simulink library "ammclib_bam_s32k14x"  (Simulink 9.0)
settings: Solver=ode45  StartTime=0.0  StopTime=10.0  RelTol=1e-3
undefined symbols (not defined in the file): f16A1, f16A2, f16B0, f16B1, f16B2, f16C1, f16CC1, f16CC1sc, f16CC1sc_D, f16CC1sc_Q, f16CC1scD, f16CC1scQ, f16CC2, f16CC2sc, f16CC2sc_D, f16CC2sc_Q, f16CC2scD, f16CC2scQ, f16DerivGain, f16EGain, f16FiltCoef, f16HystOff, f16HystOn, f16IGain, f16IntegGain, f16IntegGainFW, f16IntegGainQ, f16Kd, f16Kq, f16Limit, f16LowerLim, f16LowerLimit_D, f16LowerLimit_Q, f16ModIndex, f16OutValOff, f16OutValOn, f16PropGain, f16PropGainFW, f16PropGainQ, f16RampDown, f16RampUp, f16UGain, f16UpperLim, f16UpperLimit, f16UpperLimit_D, f16UpperLimit_Q, f16WIGain, f32A1, f32A2, f32B0, f32B1, f32B2, f32C1, f32CC1, f32CC1sc, f32CC1sc_D, f32CC1sc_Q, f32CC1scD, f32CC1scQ, f32CC2 ... (+122)
(part 5 of 11)

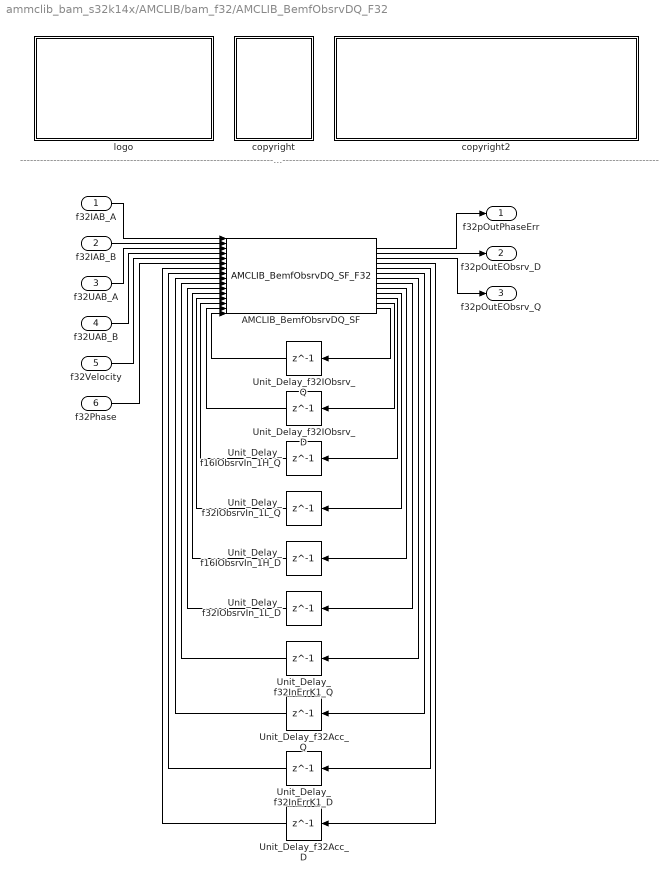
== system ammclib_bam_s32k14x/AMCLIB/bam_f32/AMCLIB_BemfObsrvDQ_F32 ==
  note: ---------------------------------------------------------------------------------------------------------------------------------------------------------------------------------------------------
  f32IAB_A : Inport
  f32IAB_B : Inport  Port=2
  f32UAB_A : Inport  Port=3
  f32UAB_B : Inport  Port=4
  f32Velocity : Inport  Port=5
  f32Phase : Inport  Port=6
  AMCLIB_BemfObsrvDQ_SF : S-Function  FunctionName=AMCLIB_BemfObsrvDQ_SF_F32  Parameters=f32IGain,f32UGain,f32WIGain,f32EGain,s16Shift,f32CC1sc_D,f32CC1sc_Q,f32CC2sc_D,f32CC2sc_Q,f32UpperLimit_D,f32UpperLimit_Q,f32LowerLimit_D,f32LowerLimit_Q,u16NShift  SFunctionDeploymentMode=off  EnableBusSupport=off
  Unit_Delay_f16IObsrvIn_1H_D : Delay  DelayLength=1  InitialCondition=0
  Unit_Delay_f16IObsrvIn_1H_Q : Delay  DelayLength=1  InitialCondition=0
  Unit_Delay_f32Acc_D : Delay  DelayLength=1  InitialCondition=0
  Unit_Delay_f32Acc_Q : Delay  DelayLength=1  InitialCondition=0
  Unit_Delay_f32IObsrvIn_1L_D : Delay  DelayLength=1  InitialCondition=0
  Unit_Delay_f32IObsrvIn_1L_Q : Delay  DelayLength=1  InitialCondition=0
  Unit_Delay_f32IObsrv_D : Delay  DelayLength=1  InitialCondition=0
  Unit_Delay_f32IObsrv_Q : Delay  DelayLength=1  InitialCondition=0
  Unit_Delay_f32InErrK1_D : Delay  DelayLength=1  InitialCondition=0
  Unit_Delay_f32InErrK1_Q : Delay  DelayLength=1  InitialCondition=0
  copyright : Subsystem
      mask Display: text(10,90,'FILE:');text(10,75,'DESRIPTION:');text(10,60,'COPYRIGHT:');text(10,45,'VERSION:');text(10,30,'DATE:')
  copyright2 : Subsystem
      mask Display: text(10,90,'AMCLIB_BemfObsrvDQ_BAM_F32.mdl');text(10,75,'PMSM back-EMF observer DQ.');text(10,60,'NXP');text(10,45,'1.0');text(10,30,'26-Oct-2016');
  logo : Subsystem
      mask Display: image(imread('logo.jpg'))
  f32pOutPhaseErr : Outport
  f32pOutEObsrv_D : Outport  Port=2
  f32pOutEObsrv_Q : Outport  Port=3
  wires:
  AMCLIB_BemfObsrvDQ_SF/3 -> f32pOutEObsrv_Q/1
  AMCLIB_BemfObsrvDQ_SF/2 -> f32pOutEObsrv_D/1
  AMCLIB_BemfObsrvDQ_SF/1 -> f32pOutPhaseErr/1
  f32Phase/1 -> AMCLIB_BemfObsrvDQ_SF/6
  f32Velocity/1 -> AMCLIB_BemfObsrvDQ_SF/5
  f32UAB_B/1 -> AMCLIB_BemfObsrvDQ_SF/4
  f32UAB_A/1 -> AMCLIB_BemfObsrvDQ_SF/3
  f32IAB_B/1 -> AMCLIB_BemfObsrvDQ_SF/2
  f32IAB_A/1 -> AMCLIB_BemfObsrvDQ_SF/1
  Unit_Delay_f32IObsrv_Q/1 -> AMCLIB_BemfObsrvDQ_SF/16
  Unit_Delay_f32IObsrv_D/1 -> AMCLIB_BemfObsrvDQ_SF/15
  Unit_Delay_f16IObsrvIn_1H_Q/1 -> AMCLIB_BemfObsrvDQ_SF/14
  AMCLIB_BemfObsrvDQ_SF/13 -> Unit_Delay_f32IObsrv_Q/1
  AMCLIB_BemfObsrvDQ_SF/12 -> Unit_Delay_f32IObsrv_D/1
  AMCLIB_BemfObsrvDQ_SF/11 -> Unit_Delay_f16IObsrvIn_1H_Q/1
  AMCLIB_BemfObsrvDQ_SF/10 -> Unit_Delay_f32IObsrvIn_1L_Q/1
  Unit_Delay_f32IObsrvIn_1L_Q/1 -> AMCLIB_BemfObsrvDQ_SF/13
  Unit_Delay_f16IObsrvIn_1H_D/1 -> AMCLIB_BemfObsrvDQ_SF/12
  AMCLIB_BemfObsrvDQ_SF/9 -> Unit_Delay_f16IObsrvIn_1H_D/1
  AMCLIB_BemfObsrvDQ_SF/8 -> Unit_Delay_f32IObsrvIn_1L_D/1
  Unit_Delay_f32IObsrvIn_1L_D/1 -> AMCLIB_BemfObsrvDQ_SF/11
  Unit_Delay_f32InErrK1_Q/1 -> AMCLIB_BemfObsrvDQ_SF/10
  AMCLIB_BemfObsrvDQ_SF/7 -> Unit_Delay_f32InErrK1_Q/1
  AMCLIB_BemfObsrvDQ_SF/6 -> Unit_Delay_f32Acc_Q/1
  Unit_Delay_f32Acc_Q/1 -> AMCLIB_BemfObsrvDQ_SF/9
  Unit_Delay_f32InErrK1_D/1 -> AMCLIB_BemfObsrvDQ_SF/8
  Unit_Delay_f32Acc_D/1 -> AMCLIB_BemfObsrvDQ_SF/7
  AMCLIB_BemfObsrvDQ_SF/5 -> Unit_Delay_f32InErrK1_D/1
  AMCLIB_BemfObsrvDQ_SF/4 -> Unit_Delay_f32Acc_D/1

== system ammclib_bam_s32k14x/AMCLIB/bam_f32/AMCLIB_CurrentLoop_F32 ==
  note: ---------------------------------------------------------------------------------------------------------------------------------------------------------------------------------------------------
  f32UDcBus : Inport
  f32IDReq : Inport  Port=2
  f32IQReq : Inport  Port=3
  f32IDFbck : Inport  Port=4
  f32IQFbck : Inport  Port=5
  AMCLIB_CurrentLoop_SF : S-Function  FunctionName=AMCLIB_CurrentLoop_SF_F32  Parameters=f32CC1scD,f32CC2scD,u16NShiftD,f32CC1scQ,f32CC2scQ,u16NShiftQ  SFunctionDeploymentMode=off  EnableBusSupport=off
  Delay{30..33} (4 alike) : Delay  DelayLength=1  InitialCondition=0
  copyright : Subsystem
      mask Display: text(10,90,'FILE:');text(10,75,'DESRIPTION:');text(10,60,'COPYRIGHT:');text(10,45,'VERSION:');text(10,30,'DATE:')
  copyright2 : Subsystem
      mask Display: text(10,90,'AMCLIB_CurrentLoop_BAM_F32.mdl');text(10,75,'PMSM Current Loop.');text(10,60,'NXP');text(10,45,'1.0');text(10,30,'25-Oct-2017');
  logo : Subsystem
      mask Display: image(imread('logo.jpg'))
  pOutUDReq : Outport
  pOutUQReq : Outport  Port=2
  wires:
  f32UDcBus/1 -> AMCLIB_CurrentLoop_SF/1
  f32IDReq/1 -> AMCLIB_CurrentLoop_SF/2
  f32IQReq/1 -> AMCLIB_CurrentLoop_SF/3
  f32IDFbck/1 -> AMCLIB_CurrentLoop_SF/4
  f32IQFbck/1 -> AMCLIB_CurrentLoop_SF/5
  Delay32/1 -> AMCLIB_CurrentLoop_SF/6
  Delay31/1 -> AMCLIB_CurrentLoop_SF/7
  Delay30/1 -> AMCLIB_CurrentLoop_SF/8
  Delay33/1 -> AMCLIB_CurrentLoop_SF/9
  AMCLIB_CurrentLoop_SF/1 -> Delay32/1
  AMCLIB_CurrentLoop_SF/2 -> Delay31/1
  AMCLIB_CurrentLoop_SF/3 -> Delay30/1
  AMCLIB_CurrentLoop_SF/4 -> Delay33/1
  AMCLIB_CurrentLoop_SF/5 -> pOutUDReq/1
  AMCLIB_CurrentLoop_SF/6 -> pOutUQReq/1

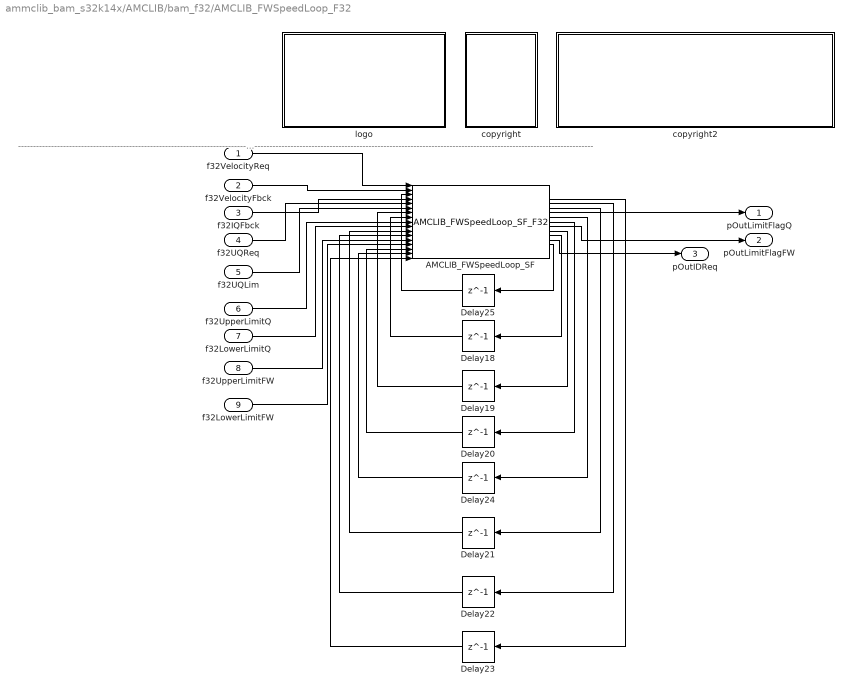
== system ammclib_bam_s32k14x/AMCLIB/bam_f32/AMCLIB_FWSpeedLoop_F32 ==
  note: ---------------------------------------------------------------------------------------------------------------------------------------------------------------------------------------------------
  f32VelocityReq : Inport
  f32VelocityFbck : Inport  Port=2
  f32IQFbck : Inport  Port=3
  f32UQReq : Inport  Port=4
  f32UQLim : Inport  Port=5
  f32UpperLimitQ : Inport  Port=6
  f32LowerLimitQ : Inport  Port=7
  f32UpperLimitFW : Inport  Port=8
  f32LowerLimitFW : Inport  Port=9
  AMCLIB_FWSpeedLoop_SF : S-Function  FunctionName=AMCLIB_FWSpeedLoop_SF_F32  Parameters=u16NSamplesW,u16NSamplesFW,f32PropGainQ,s16PropGainShiftQ,f32IntegGainQ,s16IntegGainShiftQ,f32PropGainFW,s16PropGainShiftFW,f32IntegGainFW,s16IntegGainShiftFW,f32RampUp,f32RampDown  SFunctionDeploymentMode=off  EnableBusSupport=off
  Delay{18..25} (8 alike) : Delay  DelayLength=1  InitialCondition=0
  copyright : Subsystem
      mask Display: text(10,90,'FILE:');text(10,75,'DESRIPTION:');text(10,60,'COPYRIGHT:');text(10,45,'VERSION:');text(10,30,'DATE:')
  copyright2 : Subsystem
      mask Display: text(10,90,'AMCLIB_FWSpeedLoop_BAM_F32.mdl');text(10,75,'Speed Loop with Field Weakening.');text(10,60,'NXP');text(10,45,'1.0');text(10,30,'28-Aug-2017');
  logo : Subsystem
      mask Display: image(imread('logo.jpg'))
  pOutLimitFlagQ : Outport
  pOutLimitFlagFW : Outport  Port=2
  pOutIDReq : Outport  Port=3
  wires:
  f32VelocityReq/1 -> AMCLIB_FWSpeedLoop_SF/1
  f32VelocityFbck/1 -> AMCLIB_FWSpeedLoop_SF/2
  Delay25/1 -> AMCLIB_FWSpeedLoop_SF/3
  f32IQFbck/1 -> AMCLIB_FWSpeedLoop_SF/4
  f32UQReq/1 -> AMCLIB_FWSpeedLoop_SF/5
  f32UQLim/1 -> AMCLIB_FWSpeedLoop_SF/6
  Delay19/1 -> AMCLIB_FWSpeedLoop_SF/7
  Delay18/1 -> AMCLIB_FWSpeedLoop_SF/8
  f32UpperLimitQ/1 -> AMCLIB_FWSpeedLoop_SF/9
  f32LowerLimitQ/1 -> AMCLIB_FWSpeedLoop_SF/10
  Delay21/1 -> AMCLIB_FWSpeedLoop_SF/11
  Delay22/1 -> AMCLIB_FWSpeedLoop_SF/12
  f32UpperLimitFW/1 -> AMCLIB_FWSpeedLoop_SF/13
  f32LowerLimitFW/1 -> AMCLIB_FWSpeedLoop_SF/14
  Delay20/1 -> AMCLIB_FWSpeedLoop_SF/15
  Delay24/1 -> AMCLIB_FWSpeedLoop_SF/16
  Delay23/1 -> AMCLIB_FWSpeedLoop_SF/17
  AMCLIB_FWSpeedLoop_SF/1 -> Delay23/1
  AMCLIB_FWSpeedLoop_SF/2 -> Delay22/1
  AMCLIB_FWSpeedLoop_SF/3 -> Delay21/1
  AMCLIB_FWSpeedLoop_SF/4 -> pOutLimitFlagQ/1
  AMCLIB_FWSpeedLoop_SF/5 -> Delay24/1
  AMCLIB_FWSpeedLoop_SF/6 -> Delay20/1
  AMCLIB_FWSpeedLoop_SF/7 -> pOutLimitFlagFW/1
  AMCLIB_FWSpeedLoop_SF/8 -> Delay19/1
  AMCLIB_FWSpeedLoop_SF/9 -> Delay18/1
  AMCLIB_FWSpeedLoop_SF/10 -> pOutIDReq/1
  AMCLIB_FWSpeedLoop_SF/11 -> Delay25/1

== system ammclib_bam_s32k14x/AMCLIB/bam_f32/AMCLIB_FW_F32 ==
  note: ---------------------------------------------------------------------------------------------------------------------------------------------------------------------------------------------------
  f32ReqAmp : Inport
  f32VelocityFbck : Inport  Port=2
  f32IQFbck : Inport  Port=3
  f32UQReq : Inport  Port=4
  f32UQLim : Inport  Port=5
  f32UpperLimitFW : Inport  Port=6
  f32LowerLimitFW : Inport  Port=7
  AMCLIB_FW_SF : S-Function  FunctionName=AMCLIB_FW_SF_F32  Parameters=u16NSamplesFW,f32PropGainFW,s16PropGainShiftFW,f32IntegGainFW,s16IntegGainShiftFW  SFunctionDeploymentMode=off  EnableBusSupport=off
  Delay{26..29} (4 alike) : Delay  DelayLength=1  InitialCondition=0
  copyright : Subsystem
      mask Display: text(10,90,'FILE:');text(10,75,'DESRIPTION:');text(10,60,'COPYRIGHT:');text(10,45,'VERSION:');text(10,30,'DATE:')
  copyright2 : Subsystem
      mask Display: text(10,90,'AMCLIB_FW_BAM_F32.mdl');text(10,75,'Speed Loop with Field Weakening.');text(10,60,'NXP');text(10,45,'1.0');text(10,30,'28-Aug-2017');
  logo : Subsystem
      mask Display: image(imread('logo.jpg'))
  pOutLimitFlagFW : Outport
  pOutIDReq : Outport  Port=2
  wires:
  f32ReqAmp/1 -> AMCLIB_FW_SF/1
  f32VelocityFbck/1 -> AMCLIB_FW_SF/2
  Delay29/1 -> AMCLIB_FW_SF/3
  f32IQFbck/1 -> AMCLIB_FW_SF/4
  f32UQReq/1 -> AMCLIB_FW_SF/5
  f32UQLim/1 -> AMCLIB_FW_SF/6
  Delay26/1 -> AMCLIB_FW_SF/7
  f32UpperLimitFW/1 -> AMCLIB_FW_SF/8
  f32LowerLimitFW/1 -> AMCLIB_FW_SF/9
  Delay27/1 -> AMCLIB_FW_SF/10
  Delay28/1 -> AMCLIB_FW_SF/11
  AMCLIB_FW_SF/1 -> Delay28/1
  AMCLIB_FW_SF/2 -> Delay27/1
  AMCLIB_FW_SF/3 -> pOutLimitFlagFW/1
  AMCLIB_FW_SF/4 -> Delay26/1
  AMCLIB_FW_SF/5 -> pOutIDReq/1
  AMCLIB_FW_SF/6 -> Delay29/1

== system ammclib_bam_s32k14x/AMCLIB/bam_f32/AMCLIB_SpeedLoop_F32 ==
  note: ---------------------------------------------------------------------------------------------------------------------------------------------------------------------------------------------------
  f32VelocityReq : Inport
  f32VelocityFbck : Inport  Port=2
  f32UpperLimitQ : Inport  Port=3
  f32LowerLimitQ : Inport  Port=4
  AMCLIB_SpeedLoop_SF : S-Function  FunctionName=AMCLIB_SpeedLoop_SF_F32  Parameters=u16NSamplesW,f32PropGainQ,s16PropGainShiftQ,f32IntegGainQ,s16IntegGainShiftQ,f32RampUp,f32RampDown  SFunctionDeploymentMode=off  EnableBusSupport=off
  Delay{1,14..15,17} (4 alike) : Delay  DelayLength=1  InitialCondition=0
  copyright : Subsystem
      mask Display: text(10,90,'FILE:');text(10,75,'DESRIPTION:');text(10,60,'COPYRIGHT:');text(10,45,'VERSION:');text(10,30,'DATE:')
  copyright2 : Subsystem
      mask Display: text(10,90,'AMCLIB_SpeedLoop_BAM_F32.mdl');text(10,75,'Speed Loop with Field Weakening.');text(10,60,'NXP');text(10,45,'1.0');text(10,30,'28-Aug-2017');
  logo : Subsystem
      mask Display: image(imread('logo.jpg'))
  pOutLimitFlagQ : Outport
  pOutIQReq : Outport  Port=2
  wires:
  f32VelocityReq/1 -> AMCLIB_SpeedLoop_SF/1
  f32VelocityFbck/1 -> AMCLIB_SpeedLoop_SF/2
  Delay17/1 -> AMCLIB_SpeedLoop_SF/3
  f32UpperLimitQ/1 -> AMCLIB_SpeedLoop_SF/4
  f32LowerLimitQ/1 -> AMCLIB_SpeedLoop_SF/5
  Delay14/1 -> AMCLIB_SpeedLoop_SF/6
  Delay15/1 -> AMCLIB_SpeedLoop_SF/7
  Delay1/1 -> AMCLIB_SpeedLoop_SF/8
  AMCLIB_SpeedLoop_SF/1 -> Delay1/1
  AMCLIB_SpeedLoop_SF/2 -> Delay15/1
  AMCLIB_SpeedLoop_SF/3 -> Delay14/1
  AMCLIB_SpeedLoop_SF/4 -> pOutLimitFlagQ/1
  AMCLIB_SpeedLoop_SF/5 -> Delay17/1
  AMCLIB_SpeedLoop_SF/6 -> pOutIQReq/1

== system ammclib_bam_s32k14x/AMCLIB/bam_f32/AMCLIB_TrackObsrv_F32 ==
  note: ---------------------------------------------------------------------------------------------------------------------------------------------------------------------------------------------------
  f32PhaseErr : Inport
  f32UpperLimit : Inport  Port=2
  f32LowerLimit : Inport  Port=3
  AMCLIB_TrackObsrv_SF : S-Function  FunctionName=AMCLIB_TrackObsrv_SF_F32  Parameters=f32CC1sc,f32CC2sc,u16NShift,f32C1,u16IntegNShift  SFunctionDeploymentMode=off  EnableBusSupport=off
  Unit_Delay_f32Acc : Delay  DelayLength=1  InitialCondition=0
  Unit_Delay_f32InErrK1 : Delay  DelayLength=1  InitialCondition=0
  Unit_Delay_f32InK1 : Delay  DelayLength=1  InitialCondition=0
  Unit_Delay_f32State : Delay  DelayLength=1  InitialCondition=0
  copyright : Subsystem
      mask Display: text(10,90,'FILE:');text(10,75,'DESRIPTION:');text(10,60,'COPYRIGHT:');text(10,45,'VERSION:');text(10,30,'DATE:')
  copyright2 : Subsystem
      mask Display: text(10,90,'AMCLIB_TrackObsrv_BAM_F32.mdl');text(10,75,'Tracking observer function.');text(10,60,'NXP');text(10,45,'1.0');text(10,30,'29-Jul-2016');
  logo : Subsystem
      mask Display: image(imread('logo.jpg'))
  f32PosEst : Outport
  f32VelocityEst : Outport  Port=2
  wires:
  AMCLIB_TrackObsrv_SF/2 -> f32VelocityEst/1
  AMCLIB_TrackObsrv_SF/1 -> f32PosEst/1
  f32LowerLimit/1 -> AMCLIB_TrackObsrv_SF/5
  f32UpperLimit/1 -> AMCLIB_TrackObsrv_SF/4
  f32PhaseErr/1 -> AMCLIB_TrackObsrv_SF/1
  Unit_Delay_f32InK1/1 -> AMCLIB_TrackObsrv_SF/7
  AMCLIB_TrackObsrv_SF/6 -> Unit_Delay_f32InK1/1
  Unit_Delay_f32State/1 -> AMCLIB_TrackObsrv_SF/6
  AMCLIB_TrackObsrv_SF/5 -> Unit_Delay_f32State/1
  Unit_Delay_f32InErrK1/1 -> AMCLIB_TrackObsrv_SF/3
  Unit_Delay_f32Acc/1 -> AMCLIB_TrackObsrv_SF/2
  AMCLIB_TrackObsrv_SF/4 -> Unit_Delay_f32InErrK1/1
  AMCLIB_TrackObsrv_SF/3 -> Unit_Delay_f32Acc/1

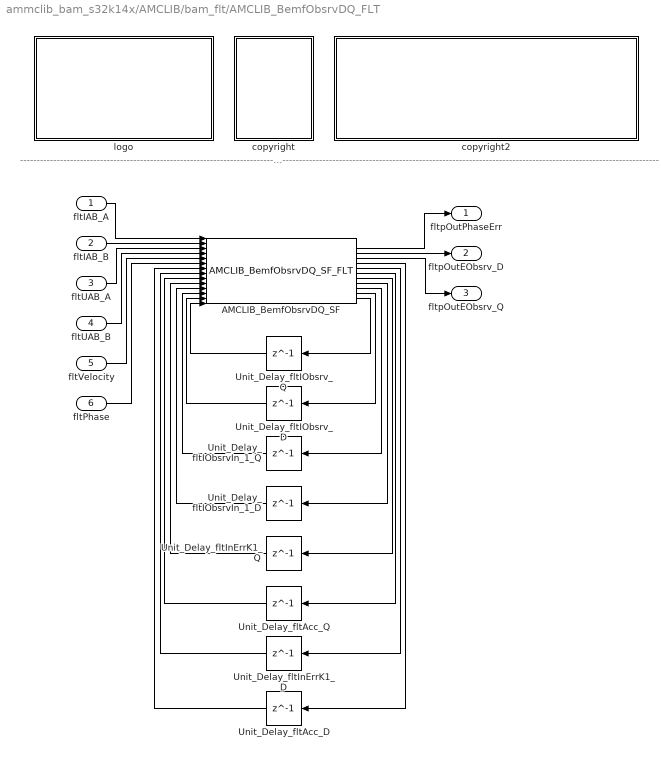
== system ammclib_bam_s32k14x/AMCLIB/bam_flt/AMCLIB_BemfObsrvDQ_FLT ==
  note: ---------------------------------------------------------------------------------------------------------------------------------------------------------------------------------------------------
  fltIAB_A : Inport
  fltIAB_B : Inport  Port=2
  fltUAB_A : Inport  Port=3
  fltUAB_B : Inport  Port=4
  fltVelocity : Inport  Port=5
  fltPhase : Inport  Port=6
  AMCLIB_BemfObsrvDQ_SF : S-Function  FunctionName=AMCLIB_BemfObsrvDQ_SF_FLT  Parameters=fltIGain,fltUGain,fltWIGain,fltEGain,fltCC1sc_D,fltCC1sc_Q,fltCC2sc_D,fltCC2sc_Q,fltUpperLimit_D,fltUpperLimit_Q,fltLowerLimit_D,fltLowerLimit_Q  SFunctionDeploymentMode=off  EnableBusSupport=off
  Unit_Delay_fltAcc_D : Delay  DelayLength=1  InitialCondition=0
  Unit_Delay_fltAcc_Q : Delay  DelayLength=1  InitialCondition=0
  Unit_Delay_fltIObsrvIn_1_D : Delay  DelayLength=1  InitialCondition=0
  Unit_Delay_fltIObsrvIn_1_Q : Delay  DelayLength=1  InitialCondition=0
  Unit_Delay_fltIObsrv_D : Delay  DelayLength=1  InitialCondition=0
  Unit_Delay_fltIObsrv_Q : Delay  DelayLength=1  InitialCondition=0
  Unit_Delay_fltInErrK1_D : Delay  DelayLength=1  InitialCondition=0
  Unit_Delay_fltInErrK1_Q : Delay  DelayLength=1  InitialCondition=0
  copyright : Subsystem
      mask Display: text(10,90,'FILE:');text(10,75,'DESRIPTION:');text(10,60,'COPYRIGHT:');text(10,45,'VERSION:');text(10,30,'DATE:')
  copyright2 : Subsystem
      mask Display: text(10,90,'AMCLIB_BemfObsrvDQ_BAM_FLT.mdl');text(10,75,'PMSM back-EMF observer DQ.');text(10,60,'NXP');text(10,45,'1.0');text(10,30,'26-Oct-2016');
  logo : Subsystem
      mask Display: image(imread('logo.jpg'))
  fltpOutPhaseErr : Outport
  fltpOutEObsrv_D : Outport  Port=2
  fltpOutEObsrv_Q : Outport  Port=3
  wires:
  AMCLIB_BemfObsrvDQ_SF/3 -> fltpOutEObsrv_Q/1
  AMCLIB_BemfObsrvDQ_SF/2 -> fltpOutEObsrv_D/1
  AMCLIB_BemfObsrvDQ_SF/1 -> fltpOutPhaseErr/1
  fltPhase/1 -> AMCLIB_BemfObsrvDQ_SF/6
  fltVelocity/1 -> AMCLIB_BemfObsrvDQ_SF/5
  fltUAB_B/1 -> AMCLIB_BemfObsrvDQ_SF/4
  fltUAB_A/1 -> AMCLIB_BemfObsrvDQ_SF/3
  fltIAB_B/1 -> AMCLIB_BemfObsrvDQ_SF/2
  fltIAB_A/1 -> AMCLIB_BemfObsrvDQ_SF/1
  Unit_Delay_fltIObsrv_Q/1 -> AMCLIB_BemfObsrvDQ_SF/14
  Unit_Delay_fltIObsrv_D/1 -> AMCLIB_BemfObsrvDQ_SF/13
  Unit_Delay_fltIObsrvIn_1_Q/1 -> AMCLIB_BemfObsrvDQ_SF/12
  Unit_Delay_fltIObsrvIn_1_D/1 -> AMCLIB_BemfObsrvDQ_SF/11
  Unit_Delay_fltInErrK1_Q/1 -> AMCLIB_BemfObsrvDQ_SF/10
  Unit_Delay_fltAcc_Q/1 -> AMCLIB_BemfObsrvDQ_SF/9
  Unit_Delay_fltInErrK1_D/1 -> AMCLIB_BemfObsrvDQ_SF/8
  Unit_Delay_fltAcc_D/1 -> AMCLIB_BemfObsrvDQ_SF/7
  AMCLIB_BemfObsrvDQ_SF/11 -> Unit_Delay_fltIObsrv_Q/1
  AMCLIB_BemfObsrvDQ_SF/10 -> Unit_Delay_fltIObsrv_D/1
  AMCLIB_BemfObsrvDQ_SF/9 -> Unit_Delay_fltIObsrvIn_1_Q/1
  AMCLIB_BemfObsrvDQ_SF/8 -> Unit_Delay_fltIObsrvIn_1_D/1
  AMCLIB_BemfObsrvDQ_SF/7 -> Unit_Delay_fltInErrK1_Q/1
  AMCLIB_BemfObsrvDQ_SF/6 -> Unit_Delay_fltAcc_Q/1
  AMCLIB_BemfObsrvDQ_SF/5 -> Unit_Delay_fltInErrK1_D/1
  AMCLIB_BemfObsrvDQ_SF/4 -> Unit_Delay_fltAcc_D/1

== system ammclib_bam_s32k14x/AMCLIB/bam_flt/AMCLIB_CurrentLoop_FLT ==
  note: ---------------------------------------------------------------------------------------------------------------------------------------------------------------------------------------------------
  fltUDcBus : Inport
  fltIDReq : Inport  Port=2
  fltIQReq : Inport  Port=3
  fltIDFbck : Inport  Port=4
  fltIQFbck : Inport  Port=5
  AMCLIB_CurrentLoop_SF : S-Function  FunctionName=AMCLIB_CurrentLoop_SF_FLT  Parameters=fltCC1scD,fltCC2scD,fltCC1scQ,fltCC2scQ  SFunctionDeploymentMode=off  EnableBusSupport=off
  Delay{28..31} (4 alike) : Delay  DelayLength=1  InitialCondition=0
  copyright : Subsystem
      mask Display: text(10,90,'FILE:');text(10,75,'DESRIPTION:');text(10,60,'COPYRIGHT:');text(10,45,'VERSION:');text(10,30,'DATE:')
  copyright2 : Subsystem
      mask Display: text(10,90,'AMCLIB_CurrentLoop_BAM_FLT.mdl');text(10,75,'PMSM Current Loop.');text(10,60,'NXP');text(10,45,'1.0');text(10,30,'25-Oct-2017');
  logo : Subsystem
      mask Display: image(imread('logo.jpg'))
  pOutUDReq : Outport
  pOutUQReq : Outport  Port=2
  wires:
  fltUDcBus/1 -> AMCLIB_CurrentLoop_SF/1
  fltIDReq/1 -> AMCLIB_CurrentLoop_SF/2
  fltIQReq/1 -> AMCLIB_CurrentLoop_SF/3
  fltIDFbck/1 -> AMCLIB_CurrentLoop_SF/4
  fltIQFbck/1 -> AMCLIB_CurrentLoop_SF/5
  Delay30/1 -> AMCLIB_CurrentLoop_SF/6
  Delay29/1 -> AMCLIB_CurrentLoop_SF/7
  Delay28/1 -> AMCLIB_CurrentLoop_SF/8
  Delay31/1 -> AMCLIB_CurrentLoop_SF/9
  AMCLIB_CurrentLoop_SF/1 -> Delay30/1
  AMCLIB_CurrentLoop_SF/2 -> Delay29/1
  AMCLIB_CurrentLoop_SF/3 -> Delay28/1
  AMCLIB_CurrentLoop_SF/4 -> Delay31/1
  AMCLIB_CurrentLoop_SF/5 -> pOutUDReq/1
  AMCLIB_CurrentLoop_SF/6 -> pOutUQReq/1

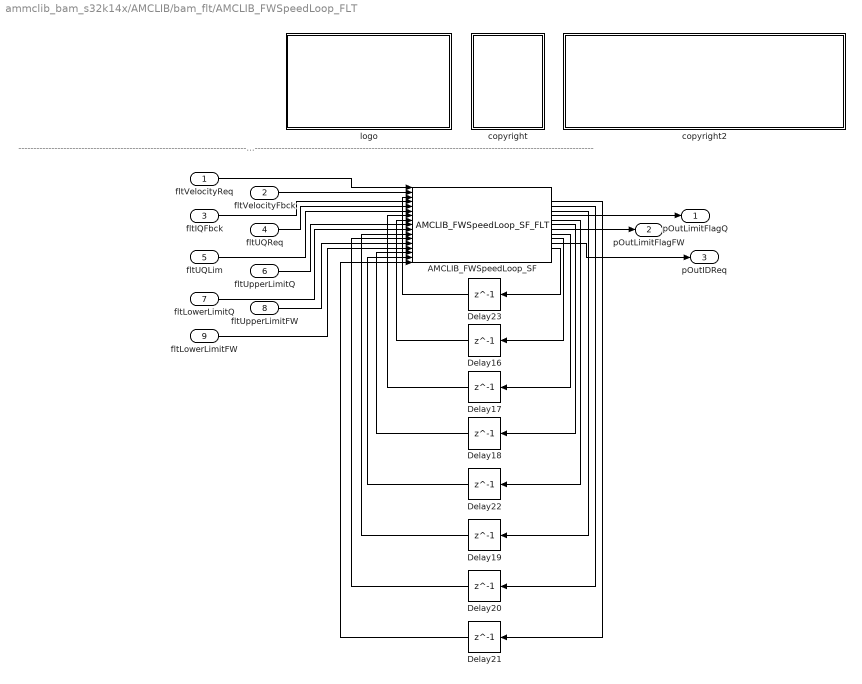
== system ammclib_bam_s32k14x/AMCLIB/bam_flt/AMCLIB_FWSpeedLoop_FLT ==
  note: ---------------------------------------------------------------------------------------------------------------------------------------------------------------------------------------------------
  fltVelocityReq : Inport
  fltVelocityFbck : Inport  Port=2
  fltIQFbck : Inport  Port=3
  fltUQReq : Inport  Port=4
  fltUQLim : Inport  Port=5
  fltUpperLimitQ : Inport  Port=6
  fltLowerLimitQ : Inport  Port=7
  fltUpperLimitFW : Inport  Port=8
  fltLowerLimitFW : Inport  Port=9
  AMCLIB_FWSpeedLoop_SF : S-Function  FunctionName=AMCLIB_FWSpeedLoop_SF_FLT  Parameters=fltLambdaW,fltLambdaFW,fltPropGainQ,fltIntegGainQ,fltPropGainFW,fltIntegGainFW,fltRampUp,fltRampDown,fltUmaxDivImax  SFunctionDeploymentMode=off  EnableBusSupport=off
  Delay{16..23} (8 alike) : Delay  DelayLength=1  InitialCondition=0
  copyright : Subsystem
      mask Display: text(10,90,'FILE:');text(10,75,'DESRIPTION:');text(10,60,'COPYRIGHT:');text(10,45,'VERSION:');text(10,30,'DATE:')
  copyright2 : Subsystem
      mask Display: text(10,90,'AMCLIB_FWSpeedLoop_BAM_FLT.mdl');text(10,75,'Speed Loop with Field Weakening.');text(10,60,'NXP');text(10,45,'1.0');text(10,30,'14-Sep-2017');
  logo : Subsystem
      mask Display: image(imread('logo.jpg'))
  pOutLimitFlagQ : Outport
  pOutLimitFlagFW : Outport  Port=2
  pOutIDReq : Outport  Port=3
  wires:
  fltVelocityReq/1 -> AMCLIB_FWSpeedLoop_SF/1
  fltVelocityFbck/1 -> AMCLIB_FWSpeedLoop_SF/2
  Delay23/1 -> AMCLIB_FWSpeedLoop_SF/3
  fltIQFbck/1 -> AMCLIB_FWSpeedLoop_SF/4
  fltUQReq/1 -> AMCLIB_FWSpeedLoop_SF/5
  fltUQLim/1 -> AMCLIB_FWSpeedLoop_SF/6
  Delay17/1 -> AMCLIB_FWSpeedLoop_SF/7
  Delay16/1 -> AMCLIB_FWSpeedLoop_SF/8
  fltUpperLimitQ/1 -> AMCLIB_FWSpeedLoop_SF/9
  fltLowerLimitQ/1 -> AMCLIB_FWSpeedLoop_SF/10
  Delay19/1 -> AMCLIB_FWSpeedLoop_SF/11
  Delay20/1 -> AMCLIB_FWSpeedLoop_SF/12
  fltUpperLimitFW/1 -> AMCLIB_FWSpeedLoop_SF/13
  fltLowerLimitFW/1 -> AMCLIB_FWSpeedLoop_SF/14
  Delay18/1 -> AMCLIB_FWSpeedLoop_SF/15
  Delay22/1 -> AMCLIB_FWSpeedLoop_SF/16
  Delay21/1 -> AMCLIB_FWSpeedLoop_SF/17
  AMCLIB_FWSpeedLoop_SF/2 -> Delay20/1
  AMCLIB_FWSpeedLoop_SF/3 -> Delay19/1
  AMCLIB_FWSpeedLoop_SF/4 -> pOutLimitFlagQ/1
  AMCLIB_FWSpeedLoop_SF/5 -> Delay22/1
  AMCLIB_FWSpeedLoop_SF/6 -> Delay18/1
  AMCLIB_FWSpeedLoop_SF/7 -> pOutLimitFlagFW/1
  AMCLIB_FWSpeedLoop_SF/8 -> Delay17/1
  AMCLIB_FWSpeedLoop_SF/9 -> Delay16/1
  AMCLIB_FWSpeedLoop_SF/10 -> pOutIDReq/1
  AMCLIB_FWSpeedLoop_SF/11 -> Delay23/1
  AMCLIB_FWSpeedLoop_SF/1 -> Delay21/1

== system ammclib_bam_s32k14x/AMCLIB/bam_flt/AMCLIB_FW_FLT ==
  note: ---------------------------------------------------------------------------------------------------------------------------------------------------------------------------------------------------
  fltReqAmp : Inport
  fltVelocityFbck : Inport  Port=2
  fltIQFbck : Inport  Port=3
  fltUQReq : Inport  Port=4
  fltUQLim : Inport  Port=5
  fltUpperLimitFW : Inport  Port=6
  fltLowerLimitFW : Inport  Port=7
  AMCLIB_FW_SF : S-Function  FunctionName=AMCLIB_FW_SF_FLT  Parameters=fltLambdaFW,fltPropGainFW,fltIntegGainFW,fltUmaxDivImax  SFunctionDeploymentMode=off  EnableBusSupport=off
  Delay{24..27} (4 alike) : Delay  DelayLength=1  InitialCondition=0
  copyright : Subsystem
      mask Display: text(10,90,'FILE:');text(10,75,'DESRIPTION:');text(10,60,'COPYRIGHT:');text(10,45,'VERSION:');text(10,30,'DATE:')
  copyright2 : Subsystem
      mask Display: text(10,90,'AMCLIB_FW_BAM_FLT.mdl');text(10,75,'Speed Loop with Field Weakening.');text(10,60,'NXP');text(10,45,'1.0');text(10,30,'14-Sep-2017');
  logo : Subsystem
      mask Display: image(imread('logo.jpg'))
  pOutLimitFlagFW : Outport
  pOutIDReq : Outport  Port=2
  wires:
  fltReqAmp/1 -> AMCLIB_FW_SF/1
  fltVelocityFbck/1 -> AMCLIB_FW_SF/2
  Delay27/1 -> AMCLIB_FW_SF/3
  fltIQFbck/1 -> AMCLIB_FW_SF/4
  fltUQReq/1 -> AMCLIB_FW_SF/5
  fltUQLim/1 -> AMCLIB_FW_SF/6
  Delay24/1 -> AMCLIB_FW_SF/7
  fltUpperLimitFW/1 -> AMCLIB_FW_SF/8
  fltLowerLimitFW/1 -> AMCLIB_FW_SF/9
  Delay25/1 -> AMCLIB_FW_SF/10
  Delay26/1 -> AMCLIB_FW_SF/11
  AMCLIB_FW_SF/1 -> Delay26/1
  AMCLIB_FW_SF/2 -> Delay25/1
  AMCLIB_FW_SF/3 -> pOutLimitFlagFW/1
  AMCLIB_FW_SF/4 -> Delay24/1
  AMCLIB_FW_SF/5 -> pOutIDReq/1
  AMCLIB_FW_SF/6 -> Delay27/1

== system ammclib_bam_s32k14x/AMCLIB/bam_flt/AMCLIB_SpeedLoop_FLT ==
  note: ---------------------------------------------------------------------------------------------------------------------------------------------------------------------------------------------------
  fltVelocityReq : Inport
  fltVelocityFbck : Inport  Port=2
  fltUpperLimitQ : Inport  Port=3
  fltLowerLimitQ : Inport  Port=4
  AMCLIB_SpeedLoop_SF : S-Function  FunctionName=AMCLIB_SpeedLoop_SF_FLT  Parameters=fltLambdaW,fltPropGainQ,fltIntegGainQ,fltRampUp,fltRampDown  SFunctionDeploymentMode=off  EnableBusSupport=off
  Delay{12..15} (4 alike) : Delay  DelayLength=1  InitialCondition=0
  copyright : Subsystem
      mask Display: text(10,90,'FILE:');text(10,75,'DESRIPTION:');text(10,60,'COPYRIGHT:');text(10,45,'VERSION:');text(10,30,'DATE:')
  copyright2 : Subsystem
      mask Display: text(10,90,'AMCLIB_SpeedLoop_BAM_FLT.mdl');text(10,75,'Speed Loop with Field Weakening.');text(10,60,'NXP');text(10,45,'1.0');text(10,30,'28-Aug-2017');
  logo : Subsystem
      mask Display: image(imread('logo.jpg'))
  pOutLimitFlagQ : Outport
  pOutIQReq : Outport  Port=2
  wires:
  fltVelocityReq/1 -> AMCLIB_SpeedLoop_SF/1
  fltVelocityFbck/1 -> AMCLIB_SpeedLoop_SF/2
  Delay12/1 -> AMCLIB_SpeedLoop_SF/3
  fltUpperLimitQ/1 -> AMCLIB_SpeedLoop_SF/4
  fltLowerLimitQ/1 -> AMCLIB_SpeedLoop_SF/5
  Delay13/1 -> AMCLIB_SpeedLoop_SF/6
  Delay14/1 -> AMCLIB_SpeedLoop_SF/7
  Delay15/1 -> AMCLIB_SpeedLoop_SF/8
  AMCLIB_SpeedLoop_SF/1 -> Delay15/1
  AMCLIB_SpeedLoop_SF/2 -> Delay14/1
  AMCLIB_SpeedLoop_SF/3 -> Delay13/1
  AMCLIB_SpeedLoop_SF/4 -> pOutLimitFlagQ/1
  AMCLIB_SpeedLoop_SF/5 -> Delay12/1
  AMCLIB_SpeedLoop_SF/6 -> pOutIQReq/1

== system ammclib_bam_s32k14x/AMCLIB/bam_flt/AMCLIB_TrackObsrv_FLT ==
  note: ---------------------------------------------------------------------------------------------------------------------------------------------------------------------------------------------------
  fltPhaseErr : Inport
  fltUpperLimit : Inport  Port=2
  fltLowerLimit : Inport  Port=3
  AMCLIB_TrackObsrv_SF : S-Function  FunctionName=AMCLIB_TrackObsrv_SF_FLT  Parameters=fltCC1,fltCC2,fltC1  SFunctionDeploymentMode=off  EnableBusSupport=off
  Unit_Delay_fltAcc : Delay  DelayLength=1  InitialCondition=0
  Unit_Delay_fltInErrK1 : Delay  DelayLength=1  InitialCondition=0
  Unit_Delay_fltInK1 : Delay  DelayLength=1  InitialCondition=0
  Unit_Delay_fltState : Delay  DelayLength=1  InitialCondition=0
  copyright : Subsystem
      mask Display: text(10,90,'FILE:');text(10,75,'DESRIPTION:');text(10,60,'COPYRIGHT:');text(10,45,'VERSION:');text(10,30,'DATE:')
  copyright2 : Subsystem
      mask Display: text(10,90,'AMCLIB_TrackObsrv_BAM_FLT.mdl');text(10,75,'Tracking observer function.');text(10,60,'NXP');text(10,45,'1.0');text(10,30,'29-Jul-2016');
  logo : Subsystem
      mask Display: image(imread('logo.jpg'))
  fltPosEst : Outport
  fltVelocityEst : Outport  Port=2
  wires:
  AMCLIB_TrackObsrv_SF/2 -> fltVelocityEst/1
  AMCLIB_TrackObsrv_SF/1 -> fltPosEst/1
  fltLowerLimit/1 -> AMCLIB_TrackObsrv_SF/5
  fltUpperLimit/1 -> AMCLIB_TrackObsrv_SF/4
  fltPhaseErr/1 -> AMCLIB_TrackObsrv_SF/1
  Unit_Delay_fltInK1/1 -> AMCLIB_TrackObsrv_SF/7
  Unit_Delay_fltState/1 -> AMCLIB_TrackObsrv_SF/6
  AMCLIB_TrackObsrv_SF/6 -> Unit_Delay_fltInK1/1
  AMCLIB_TrackObsrv_SF/5 -> Unit_Delay_fltState/1
  Unit_Delay_fltInErrK1/1 -> AMCLIB_TrackObsrv_SF/3
  Unit_Delay_fltAcc/1 -> AMCLIB_TrackObsrv_SF/2
  AMCLIB_TrackObsrv_SF/4 -> Unit_Delay_fltInErrK1/1
  AMCLIB_TrackObsrv_SF/3 -> Unit_Delay_fltAcc/1

== system ammclib_bam_s32k14x/GDFLIB/bam_f16/GDFLIB_FilterFIR_F16 ==
  note: ---------------------------------------------------------------------------------------------------------------------------------------------------------------------------------------------------
  f16In : Inport
  GDFLIB_FilterFIR_SF : S-Function  FunctionName=GDFLIB_FilterFIR_SF_F16  Parameters=u16Order,pf16CoefBuf  SFunctionDeploymentMode=off  EnableBusSupport=off
  Unit Delay_pf16InBuf : UnitDelay  SampleTime=-1
  Unit_Delay_u16InIdx : UnitDelay  SampleTime=-1
  copyright : Subsystem
      mask Display:
      | text(10,90,'FILE:');text(10,75,'DESRIPTION:')
      | text(10,60,'COPYRIGHT:')
      | text(10,45,'VERSION:')
      | text(10,30,'DATE:')
  copyright2 : Subsystem
      mask Display:
      | text(10,90,'GDFLIB_FilterFIR_BAM_F16.mdl');text(10,75,'FIR filter.');text(10,60,'NXP')
      | text(10,45,'0.1');text(10,30,'20-Sep-2011');
  logo : Subsystem
      mask Display: image(imread('logo.jpg'))
  f16Out : Outport
  wires:
  GDFLIB_FilterFIR_SF/1 -> f16Out/1
  f16In/1 -> GDFLIB_FilterFIR_SF/1
  Unit Delay_pf16InBuf/1 -> GDFLIB_FilterFIR_SF/3
  Unit_Delay_u16InIdx/1 -> GDFLIB_FilterFIR_SF/2
  GDFLIB_FilterFIR_SF/3 -> Unit Delay_pf16InBuf/1
  GDFLIB_FilterFIR_SF/2 -> Unit_Delay_u16InIdx/1

== system ammclib_bam_s32k14x/GDFLIB/bam_f16/GDFLIB_FilterIIR1_F16 ==
  note: ---------------------------------------------------------------------------------------------------------------------------------------------------------------------------------------------------
  f16In : Inport
  GDFLIB_FilterIIR1_SF_F16 : S-Function  FunctionName=GDFLIB_FilterIIR1_SF_F16  Parameters=f16B0,f16B1,f16A1  SFunctionDeploymentMode=off  EnableBusSupport=off
  "Unit_Delay_f16InFiltBufferX " : UnitDelay  SampleTime=-1
  Unit_Delay_f32InFiltBufferY : UnitDelay  SampleTime=-1
  copyright : Subsystem
      mask Display:
      | text(10,90,'FILE:');text(10,75,'DESRIPTION:')
      | text(10,60,'COPYRIGHT:')
      | text(10,45,'VERSION:')
      | text(10,30,'DATE:')
      | text(10,15,'AUTHOR:')
  copyright2 : Subsystem
      mask Display:
      | text(10,90,'GDFLIB_FilterIIR1_BAM_F16.mdl');text(10,75,'Direct form I first order IIR filter.');text(10,60,'NXP')
      | text(10,45,'0.1');text(10,30,'08-Apr-2014');text(10,15,'');
  logo : Subsystem
      mask Display: image(imread('logo.jpg'))
  f16Out : Outport
  wires:
  GDFLIB_FilterIIR1_SF_F16/1 -> f16Out/1
  f16In/1 -> GDFLIB_FilterIIR1_SF_F16/1
  Unit_Delay_f32InFiltBufferY/1 -> GDFLIB_FilterIIR1_SF_F16/3
  "Unit_Delay_f16InFiltBufferX "/1 -> GDFLIB_FilterIIR1_SF_F16/2
  GDFLIB_FilterIIR1_SF_F16/3 -> Unit_Delay_f32InFiltBufferY/1
  GDFLIB_FilterIIR1_SF_F16/2 -> "Unit_Delay_f16InFiltBufferX "/1

== system ammclib_bam_s32k14x/GDFLIB/bam_f16/GDFLIB_FilterIIR2_F16 ==
  note: ---------------------------------------------------------------------------------------------------------------------------------------------------------------------------------------------------
  f16In : Inport
  " Unit_Delay_f16InFiltBufferX[1] " : UnitDelay  SampleTime=-1
  " Unit_Delay_f16InFiltBufferX[2]" : UnitDelay  SampleTime=-1
  GDFLIB_FilterIIR2_SF_F16 : S-Function  FunctionName=GDFLIB_FilterIIR2_SF_F16  Parameters=f16B0,f16B1,f16B2,f16A1,f16A2  SFunctionDeploymentMode=off  EnableBusSupport=off
  Unit_Delay_f32InFiltBufferY[1] : UnitDelay  SampleTime=-1
  Unit_Delay_f32InFiltBufferY[2] : UnitDelay  SampleTime=-1
  copyright : Subsystem
      mask Display:
      | text(10,90,'FILE:');text(10,75,'DESRIPTION:')
      | text(10,60,'COPYRIGHT:')
      | text(10,45,'VERSION:')
      | text(10,30,'DATE:')
      | text(10,15,'AUTHOR:')
  copyright2 : Subsystem
      mask Display:
      | text(10,90,'GDFLIB_FilterIIR2_BAM_F16.mdl');text(10,75,'Direct form I first order IIR filter.');text(10,60,'NXP')
      | text(10,45,'0.1');text(10,30,'08-Apr-2014');text(10,15,'');
  logo : Subsystem
      mask Display: image(imread('logo.jpg'))
  f16Out : Outport
  wires:
  GDFLIB_FilterIIR2_SF_F16/1 -> f16Out/1
  f16In/1 -> GDFLIB_FilterIIR2_SF_F16/1
  GDFLIB_FilterIIR2_SF_F16/5 -> Unit_Delay_f32InFiltBufferY[2]/1
  Unit_Delay_f32InFiltBufferY[2]/1 -> GDFLIB_FilterIIR2_SF_F16/5
  Unit_Delay_f32InFiltBufferY[1]/1 -> GDFLIB_FilterIIR2_SF_F16/4
  GDFLIB_FilterIIR2_SF_F16/4 -> Unit_Delay_f32InFiltBufferY[1]/1
  GDFLIB_FilterIIR2_SF_F16/3 -> " Unit_Delay_f16InFiltBufferX[2]"/1
  " Unit_Delay_f16InFiltBufferX[2]"/1 -> GDFLIB_FilterIIR2_SF_F16/3
  " Unit_Delay_f16InFiltBufferX[1] "/1 -> GDFLIB_FilterIIR2_SF_F16/2
  GDFLIB_FilterIIR2_SF_F16/2 -> " Unit_Delay_f16InFiltBufferX[1] "/1

== system ammclib_bam_s32k14x/GDFLIB/bam_f16/GDFLIB_FilterMA_F16 ==
  note: ---------------------------------------------------------------------------------------------------------------------------------------------------------------------------------------------------
  f16In : Inport
  GDFLIB_FilterMA_SF : S-Function  FunctionName=GDFLIB_FilterMA_SF_F16  Parameters=u16NSamples  SFunctionDeploymentMode=off  EnableBusSupport=off
  Unit_Delay_f32InAcc : UnitDelay  SampleTime=-1
  copyright : Subsystem
      mask Display:
      | text(10,90,'FILE:');text(10,75,'DESRIPTION:')
      | text(10,60,'COPYRIGHT:')
      | text(10,45,'VERSION:')
      | text(10,30,'DATE:')
  copyright2 : Subsystem
      mask Display:
      | text(10,90,'GDFLIB_FilterMA_BAM_F16.mdl');text(10,75,'Recursive form moving average filter.');text(10,60,'NXP')
      | text(10,45,'0.1');text(10,30,'16-Jan-2012');
  logo : Subsystem
      mask Display: image(imread('logo.jpg'))
  f16Out : Outport
  wires:
  GDFLIB_FilterMA_SF/1 -> f16Out/1
  f16In/1 -> GDFLIB_FilterMA_SF/1
  GDFLIB_FilterMA_SF/2 -> Unit_Delay_f32InAcc/1
  Unit_Delay_f32InAcc/1 -> GDFLIB_FilterMA_SF/2

== system ammclib_bam_s32k14x/GDFLIB/bam_f32/GDFLIB_FilterFIR_F32 ==
  note: ---------------------------------------------------------------------------------------------------------------------------------------------------------------------------------------------------
  f32In : Inport
  GDFLIB_FilterFIR_SF : S-Function  FunctionName=GDFLIB_FilterFIR_SF_F32  Parameters=u32Order,pf32CoefBuf  SFunctionDeploymentMode=off  EnableBusSupport=off
  Unit Delay_pf32InBuf : UnitDelay  SampleTime=-1
  Unit_Delay_u16InIdx : UnitDelay  SampleTime=-1
  copyright : Subsystem
      mask Display:
      | text(10,90,'FILE:');text(10,75,'DESRIPTION:')
      | text(10,60,'COPYRIGHT:')
      | text(10,45,'VERSION:')
      | text(10,30,'DATE:')
  copyright2 : Subsystem
      mask Display:
      | text(10,90,'GDFLIB_FilterFIR_BAM_F32.mdl');text(10,75,'FIR filter.');text(10,60,'NXP')
      | text(10,45,'0.1');text(10,30,'20-Sep-2011');
  logo : Subsystem
      mask Display: image(imread('logo.jpg'))
  f32Out : Outport
  wires:
  GDFLIB_FilterFIR_SF/1 -> f32Out/1
  f32In/1 -> GDFLIB_FilterFIR_SF/1
  GDFLIB_FilterFIR_SF/3 -> Unit Delay_pf32InBuf/1
  GDFLIB_FilterFIR_SF/2 -> Unit_Delay_u16InIdx/1
  Unit Delay_pf32InBuf/1 -> GDFLIB_FilterFIR_SF/3
  Unit_Delay_u16InIdx/1 -> GDFLIB_FilterFIR_SF/2

== system ammclib_bam_s32k14x/GDFLIB/bam_f32/GDFLIB_FilterIIR1_F32 ==
  note: ---------------------------------------------------------------------------------------------------------------------------------------------------------------------------------------------------
  f32In : Inport
  GDFLIB_FilterIIR1_SF_F32 : S-Function  FunctionName=GDFLIB_FilterIIR1_SF_F32  Parameters=f32B0,f32B1,f32A1  SFunctionDeploymentMode=off  EnableBusSupport=off
  "Unit_Delay_f32InFiltBufferX " : UnitDelay  SampleTime=-1
  Unit_Delay_f32InFiltBufferY : UnitDelay  SampleTime=-1
  copyright : Subsystem
      mask Display:
      | text(10,90,'FILE:');text(10,75,'DESRIPTION:')
      | text(10,60,'COPYRIGHT:')
      | text(10,45,'VERSION:')
      | text(10,30,'DATE:')
      | text(10,15,'AUTHOR:')
  copyright2 : Subsystem
      mask Display:
      | text(10,90,'GDFLIB_FilterIIR1_BAM_F32.mdl');text(10,75,'Direct form I first order IIR filter.');text(10,60,'NXP')
      | text(10,45,'0.1');text(10,30,'08-Apr-2014');
  logo : Subsystem
      mask Display: image(imread('logo.jpg'))
  f32Out : Outport
  wires:
  GDFLIB_FilterIIR1_SF_F32/1 -> f32Out/1
  f32In/1 -> GDFLIB_FilterIIR1_SF_F32/1
  GDFLIB_FilterIIR1_SF_F32/3 -> Unit_Delay_f32InFiltBufferY/1
  GDFLIB_FilterIIR1_SF_F32/2 -> "Unit_Delay_f32InFiltBufferX "/1
  Unit_Delay_f32InFiltBufferY/1 -> GDFLIB_FilterIIR1_SF_F32/3
  "Unit_Delay_f32InFiltBufferX "/1 -> GDFLIB_FilterIIR1_SF_F32/2

== system ammclib_bam_s32k14x/GDFLIB/bam_f32/GDFLIB_FilterIIR2_F32 ==
  note: ---------------------------------------------------------------------------------------------------------------------------------------------------------------------------------------------------
  f32In : Inport
  " Unit_Delay_f32InFiltBufferX[1] " : UnitDelay  SampleTime=-1
  " Unit_Delay_f32InFiltBufferX[2]" : UnitDelay  SampleTime=-1
  GDFLIB_FilterIIR2_SF_F32 : S-Function  FunctionName=GDFLIB_FilterIIR2_SF_F32  Parameters=f32B0,f32B1,f32B2,f32A1,f32A2  SFunctionDeploymentMode=off  EnableBusSupport=off
  Unit_Delay_f32InFiltBufferY[1] : UnitDelay  SampleTime=-1
  Unit_Delay_f32InFiltBufferY[2] : UnitDelay  SampleTime=-1
  copyright : Subsystem
      mask Display:
      | text(10,90,'FILE:');text(10,75,'DESRIPTION:')
      | text(10,60,'COPYRIGHT:')
      | text(10,45,'VERSION:')
      | text(10,30,'DATE:')
      | text(10,15,'AUTHOR:')
  copyright2 : Subsystem
      mask Display:
      | text(10,90,'GDFLIB_FilterIIR2_BAM_F32.mdl');text(10,75,'Direct form I second order IIR filter.');text(10,60,'NXP')
      | text(10,45,'0.1');text(10,30,'08-Apr-2014');text(10,15,'');
  logo : Subsystem
      mask Display: image(imread('logo.jpg'))
  f32Out : Outport
  wires:
  GDFLIB_FilterIIR2_SF_F32/1 -> f32Out/1
  f32In/1 -> GDFLIB_FilterIIR2_SF_F32/1
  Unit_Delay_f32InFiltBufferY[2]/1 -> GDFLIB_FilterIIR2_SF_F32/5
  Unit_Delay_f32InFiltBufferY[1]/1 -> GDFLIB_FilterIIR2_SF_F32/4
  " Unit_Delay_f32InFiltBufferX[2]"/1 -> GDFLIB_FilterIIR2_SF_F32/3
  " Unit_Delay_f32InFiltBufferX[1] "/1 -> GDFLIB_FilterIIR2_SF_F32/2
  GDFLIB_FilterIIR2_SF_F32/5 -> Unit_Delay_f32InFiltBufferY[2]/1
  GDFLIB_FilterIIR2_SF_F32/4 -> Unit_Delay_f32InFiltBufferY[1]/1
  GDFLIB_FilterIIR2_SF_F32/3 -> " Unit_Delay_f32InFiltBufferX[2]"/1
  GDFLIB_FilterIIR2_SF_F32/2 -> " Unit_Delay_f32InFiltBufferX[1] "/1

== system ammclib_bam_s32k14x/GDFLIB/bam_f32/GDFLIB_FilterMA_F32 ==
  note: ---------------------------------------------------------------------------------------------------------------------------------------------------------------------------------------------------
  f32In : Inport
  GDFLIB_FilterMA_SF : S-Function  FunctionName=GDFLIB_FilterMA_SF_F32  Parameters=u16NSamples  SFunctionDeploymentMode=off  EnableBusSupport=off
  Unit_Delay_f32InAcc : UnitDelay  SampleTime=-1
  copyright : Subsystem
      mask Display:
      | text(10,90,'FILE:');text(10,75,'DESRIPTION:')
      | text(10,60,'COPYRIGHT:')
      | text(10,45,'VERSION:')
      | text(10,30,'DATE:')
  copyright2 : Subsystem
      mask Display:
      | text(10,90,'GDFLIB_FilterMA_BAM_F32.mdl');text(10,75,'Recursive form moving average filter.');text(10,60,'NXP')
      | text(10,45,'0.1');text(10,30,'16-Jan-2012');
  logo : Subsystem
      mask Display: image(imread('logo.jpg'))
  f32Out : Outport
  wires:
  GDFLIB_FilterMA_SF/1 -> f32Out/1
  f32In/1 -> GDFLIB_FilterMA_SF/1
  GDFLIB_FilterMA_SF/2 -> Unit_Delay_f32InAcc/1
  Unit_Delay_f32InAcc/1 -> GDFLIB_FilterMA_SF/2

== system ammclib_bam_s32k14x/GDFLIB/bam_flt/GDFLIB_FilterFIR_FLT ==
  note: ---------------------------------------------------------------------------------------------------------------------------------------------------------------------------------------------------
  fltIn : Inport
  GDFLIB_FilterFIR_SF : S-Function  FunctionName=GDFLIB_FilterFIR_SF_FLT  Parameters=u32Order,pfltCoefBuf  SFunctionDeploymentMode=off  EnableBusSupport=off
  Unit_Delay_pfltInBuf : UnitDelay  SampleTime=-1
  Unit_Delay_u16InIdx : UnitDelay  SampleTime=-1
  copyright : Subsystem
      mask Display:
      | text(10,90,'FILE:');text(10,75,'DESRIPTION:')
      | text(10,60,'COPYRIGHT:')
      | text(10,45,'VERSION:')
      | text(10,30,'DATE:')
  copyright2 : Subsystem
      mask Display:
      | text(10,90,'GDFLIB_FilterFIR_BAM_FLT.mdl');text(10,75,'FIR filter.');text(10,60,'NXP')
      | text(10,45,'0.1');text(10,30,'20-Sep-2011');
  logo : Subsystem
      mask Display: image(imread('logo.jpg'))
  fltOut : Outport
  wires:
  GDFLIB_FilterFIR_SF/1 -> fltOut/1
  fltIn/1 -> GDFLIB_FilterFIR_SF/1
  GDFLIB_FilterFIR_SF/3 -> Unit_Delay_pfltInBuf/1
  GDFLIB_FilterFIR_SF/2 -> Unit_Delay_u16InIdx/1
  Unit_Delay_pfltInBuf/1 -> GDFLIB_FilterFIR_SF/3
  Unit_Delay_u16InIdx/1 -> GDFLIB_FilterFIR_SF/2

== system ammclib_bam_s32k14x/GDFLIB/bam_flt/GDFLIB_FilterIIR1_FLT ==
  note: ---------------------------------------------------------------------------------------------------------------------------------------------------------------------------------------------------
  fltIn : Inport
  GDFLIB_FilterIIR1_SF_FLT : S-Function  FunctionName=GDFLIB_FilterIIR1_SF_FLT  Parameters=fltB0,fltB1,fltA1  SFunctionDeploymentMode=off  EnableBusSupport=off
  Unit_Delay _fltInFiltBufferX : UnitDelay  SampleTime=-1
  Unit_Delay_fltInFiltBufferY : UnitDelay  SampleTime=-1
  copyright : Subsystem
      mask Display:
      | text(10,90,'FILE:');text(10,75,'DESRIPTION:')
      | text(10,60,'COPYRIGHT:')
      | text(10,45,'VERSION:')
      | text(10,30,'DATE:')
      | text(10,15,'AUTHOR:')
  copyright2 : Subsystem
      mask Display:
      | text(10,90,'GDFLIB_FilterIIR1_BAM_FLT.mdl');text(10,75,'Direct form I first order IIR filter.');text(10,60,'NXP')
      | text(10,45,'0.1');text(10,30,'08-Apr-2014');text(10,15,'');
  logo : Subsystem
      mask Display: image(imread('logo.jpg'))
  fltOut : Outport
  wires:
  GDFLIB_FilterIIR1_SF_FLT/1 -> fltOut/1
  fltIn/1 -> GDFLIB_FilterIIR1_SF_FLT/1
  GDFLIB_FilterIIR1_SF_FLT/3 -> Unit_Delay_fltInFiltBufferY/1
  GDFLIB_FilterIIR1_SF_FLT/2 -> Unit_Delay _fltInFiltBufferX/1
  Unit_Delay_fltInFiltBufferY/1 -> GDFLIB_FilterIIR1_SF_FLT/3
  Unit_Delay _fltInFiltBufferX/1 -> GDFLIB_FilterIIR1_SF_FLT/2

== system ammclib_bam_s32k14x/GDFLIB/bam_flt/GDFLIB_FilterIIR2_FLT ==
  note: ---------------------------------------------------------------------------------------------------------------------------------------------------------------------------------------------------
  fltIn : Inport
  " Unit_Delay_fltInFiltBufferX[1] " : UnitDelay  SampleTime=-1
  " Unit_Delay_fltInFiltBufferX[2]" : UnitDelay  SampleTime=-1
  GDFLIB_FilterIIR2_SF_FLT : S-Function  FunctionName=GDFLIB_FilterIIR2_SF_FLT  Parameters=fltB0,fltB1,fltB2,fltA1,fltA2  SFunctionDeploymentMode=off  EnableBusSupport=off
  "Unit_Delay_fltInFiltBufferY[1] " : UnitDelay  SampleTime=-1
  Unit_Delay_fltInFiltBufferY[2] : UnitDelay  SampleTime=-1
  copyright : Subsystem
      mask Display:
      | text(10,90,'FILE:');text(10,75,'DESRIPTION:')
      | text(10,60,'COPYRIGHT:')
      | text(10,45,'VERSION:')
      | text(10,30,'DATE:')
      | text(10,15,'AUTHOR:')
  copyright2 : Subsystem
      mask Display:
      | text(10,90,'GDFLIB_FilterIIR2_BAM_FLT.mdl');text(10,75,'Direct form I second order IIR filter.');text(10,60,'NXP')
      | text(10,45,'0.1');text(10,30,'08-Apr-2014');text(10,15,'');
  logo : Subsystem
      mask Display: image(imread('logo.jpg'))
  fltOut : Outport
  wires:
  GDFLIB_FilterIIR2_SF_FLT/1 -> fltOut/1
  fltIn/1 -> GDFLIB_FilterIIR2_SF_FLT/1
  Unit_Delay_fltInFiltBufferY[2]/1 -> GDFLIB_FilterIIR2_SF_FLT/5
  "Unit_Delay_fltInFiltBufferY[1] "/1 -> GDFLIB_FilterIIR2_SF_FLT/4
  " Unit_Delay_fltInFiltBufferX[2]"/1 -> GDFLIB_FilterIIR2_SF_FLT/3
  " Unit_Delay_fltInFiltBufferX[1] "/1 -> GDFLIB_FilterIIR2_SF_FLT/2
  GDFLIB_FilterIIR2_SF_FLT/5 -> Unit_Delay_fltInFiltBufferY[2]/1
  GDFLIB_FilterIIR2_SF_FLT/4 -> "Unit_Delay_fltInFiltBufferY[1] "/1
  GDFLIB_FilterIIR2_SF_FLT/3 -> " Unit_Delay_fltInFiltBufferX[2]"/1
  GDFLIB_FilterIIR2_SF_FLT/2 -> " Unit_Delay_fltInFiltBufferX[1] "/1

== system ammclib_bam_s32k14x/GDFLIB/bam_flt/GDFLIB_FilterMA_FLT ==
  note: ---------------------------------------------------------------------------------------------------------------------------------------------------------------------------------------------------
  fltIn : Inport
  GDFLIB_FilterMA_SF : S-Function  FunctionName=GDFLIB_FilterMA_SF_FLT  Parameters=fltLambda  SFunctionDeploymentMode=off  EnableBusSupport=off
  Unit_Delay_fltInAcc : UnitDelay  SampleTime=-1
  copyright : Subsystem
      mask Display:
      | text(10,90,'FILE:');text(10,75,'DESRIPTION:')
      | text(10,60,'COPYRIGHT:')
      | text(10,45,'VERSION:')
      | text(10,30,'DATE:')
  copyright2 : Subsystem
      mask Display:
      | text(10,90,'GDFLIB_FilterMA_BAM_FLT.mdl');text(10,75,'Recursive form moving average filter.');text(10,60,'NXP')
      | text(10,45,'0.1');text(10,30,'16-Jan-2012');
  logo : Subsystem
      mask Display: image(imread('logo.jpg'))
  fltOut : Outport
  wires:
  GDFLIB_FilterMA_SF/1 -> fltOut/1
  fltIn/1 -> GDFLIB_FilterMA_SF/1
  GDFLIB_FilterMA_SF/2 -> Unit_Delay_fltInAcc/1
  Unit_Delay_fltInAcc/1 -> GDFLIB_FilterMA_SF/2

== system ammclib_bam_s32k14x/GFLIB/bam_f16/GFLIB_Acos_F16 ==
  note: ---------------------------------------------------------------------------------------------------------------------------------------------------------------------------------------------------
  f16In : Inport
  GFLIB_Acos_SF : S-Function  FunctionName=GFLIB_Acos_SF_F16  SFunctionDeploymentMode=off  EnableBusSupport=off
  copyright : Subsystem
      mask Display:
      | text(10,90,'FILE:');text(10,75,'DESRIPTION:')
      | text(10,60,'COPYRIGHT:')
      | text(10,45,'VERSION:')
      | text(10,30,'DATE:')
  copyright2 : Subsystem
      mask Display:
      | text(10,90,'GFLIB_Acos_BAM_F16.mdl');text(10,75,'Inverse cosine transformation');text(10,60,'Freescale')
      | text(10,45,'0.1');text(10,30,'31-Aug-2011');
  logo : Subsystem
      mask Display: image(imread('logo.jpg'))
  f16Out : Outport
  wires:
  GFLIB_Acos_SF/1 -> f16Out/1
  f16In/1 -> GFLIB_Acos_SF/1

== system ammclib_bam_s32k14x/GFLIB/bam_f16/GFLIB_Asin_F16 ==
  note: ---------------------------------------------------------------------------------------------------------------------------------------------------------------------------------------------------
  f16In : Inport
  GFLIB_Asin_SF : S-Function  FunctionName=GFLIB_Asin_SF_F16  SFunctionDeploymentMode=off  EnableBusSupport=off
  copyright : Subsystem
      mask Display:
      | text(10,90,'FILE:');text(10,75,'DESRIPTION:')
      | text(10,60,'COPYRIGHT:')
      | text(10,45,'VERSION:')
      | text(10,30,'DATE:')
  copyright2 : Subsystem
      mask Display:
      | text(10,90,'GFLIB_Asin_BAM_F16.mdl');text(10,75,'Inverse cosine transformation');text(10,60,'Freescale')
      | text(10,45,'0.1');text(10,30,'01-Sep-2011');
  logo : Subsystem
      mask Display: image(imread('logo.jpg'))
  f16Out : Outport
  wires:
  GFLIB_Asin_SF/1 -> f16Out/1
  f16In/1 -> GFLIB_Asin_SF/1

== system ammclib_bam_s32k14x/GFLIB/bam_f16/GFLIB_AtanYXShifted_F16 ==
  note: ---------------------------------------------------------------------------------------------------------------------------------------------------------------------------------------------------
  f16InY : Inport
  f16InX : Inport  Port=2
  GFLIB_AtanYXShifted_SF : S-Function  FunctionName=GFLIB_AtanYXShifted_SF_F16  Parameters=Ky,Kx,Ny,Nx,ThetaAdj  SFunctionDeploymentMode=off  EnableBusSupport=off
  copyright : Subsystem
      mask Display:
      | text(10,90,'FILE:');text(10,75,'DESRIPTION:')
      | text(10,60,'COPYRIGHT:')
      | text(10,45,'VERSION:')
      | text(10,30,'DATE:')
  copyright2 : Subsystem
      mask Display:
      | text(10,90,'GFLIB_AtanYXShifted_BAM_F16.mdl');text(10,75,'Shifted YX Arctangent of argument.');text(10,60,'NXP')
      | text(10,45,'0.1');text(10,30,'06-Sep-2011');
  logo : Subsystem
      mask Display: image(imread('logo.jpg'))
  f16Out : Outport
  wires:
  GFLIB_AtanYXShifted_SF/1 -> f16Out/1
  f16InX/1 -> GFLIB_AtanYXShifted_SF/2
  f16InY/1 -> GFLIB_AtanYXShifted_SF/1

== system ammclib_bam_s32k14x/GFLIB/bam_f16/GFLIB_AtanYX_F16 ==
  note: ---------------------------------------------------------------------------------------------------------------------------------------------------------------------------------------------------
  f16InY : Inport
  f16InX : Inport  Port=2
  GFLIB_AtanYX_SF : S-Function  FunctionName=GFLIB_AtanYX_SF_F16  SFunctionDeploymentMode=off  EnableBusSupport=off
  copyright : Subsystem
      mask Display:
      | text(10,90,'FILE:');text(10,75,'DESRIPTION:')
      | text(10,60,'COPYRIGHT:')
      | text(10,45,'VERSION:')
      | text(10,30,'DATE:')
  copyright2 : Subsystem
      mask Display:
      | text(10,90,'GFLIB_AtanYX_BAM_F16.mdl');text(10,75,'YX Arctangent of argument.');text(10,60,'Freescale')
      | text(10,45,'0.1');text(10,30,'05-Sep-2011');
  logo : Subsystem
      mask Display: image(imread('logo.jpg'))
  f16Out : Outport
  wires:
  GFLIB_AtanYX_SF/1 -> f16Out/1
  f16InX/1 -> GFLIB_AtanYX_SF/2
  f16InY/1 -> GFLIB_AtanYX_SF/1

== system ammclib_bam_s32k14x/GFLIB/bam_f16/GFLIB_Atan_F16 ==
  note: ---------------------------------------------------------------------------------------------------------------------------------------------------------------------------------------------------
  f16In : Inport
  GFLIB_Atan_SF : S-Function  FunctionName=GFLIB_Atan_SF_F16  SFunctionDeploymentMode=off  EnableBusSupport=off
  copyright : Subsystem
      mask Display:
      | text(10,90,'FILE:');text(10,75,'DESRIPTION:')
      | text(10,60,'COPYRIGHT:')
      | text(10,45,'VERSION:')
      | text(10,30,'DATE:')
  copyright2 : Subsystem
      mask Display:
      | text(10,90,'GFLIB_Atan_BAM_F16.mdl');text(10,75,'Inverse tangent transformation');text(10,60,'Freescale')
      | text(10,45,'0.1');text(10,30,'01-Sep-2011');
  logo : Subsystem
      mask Display: image(imread('logo.jpg'))
  f16Out : Outport
  wires:
  GFLIB_Atan_SF/1 -> f16Out/1
  f16In/1 -> GFLIB_Atan_SF/1
